simulink model "nonlinear_inverted_pendulum_simulation_direct"  (R2016b)
settings: Solver=ode15s  StartTime=0.0  StopTime=10.0  RelTol=1e-3
values from neighbouring files (symbols this model uses):
  A = sys.A    [LoopGain.m]    (also in dcontrold_dir.m = sys_d.A; main.m = [                   0,                                      ; simulation.m)
  B = sys.B    [LoopGain.m]    (also in dcontrold_dir.m = sys_d.B; main.m = [                   0; ( 3*Km*Vs)/(LinkMass*(LinkLength^2)*R; simulation.m)
  b_motor = 0    [main.m]
  C = sys.C    [LoopGain.m]    (also in dcontrold_dir.m = sys_d.C; main.m = [                   1,                                      ; simulation.m)
  g = 9.81    [main.m]
  J_total = 3.97396e-05    [InvPendModel.mat]    (also in main.m = 0.080955181411)
  K = place(A,B,Kp)    [dcontrold_dir.m]    (also in dcontrold_ind.m = place(A, B, desFbPoles); sysStateEstimatorFeedbackWithModel.m = Kaug(1:nStates))
  Kb = Km    (= 0.0265805280355)    [main.m]
  Km = Vs/kappa_id    (= 0.0265805280355)    [main.m]    (also in sysStateEstimatorFeedbackWithModel.m = Kaug(nStates + 1:end))
  L = place(A',C',Lp)'    [dcontrold_dir.m]    (also in dcontrold_ind.m = place(A', C', desObsPoles).')
  L_motor = 0.24E-3    (= 0.00024)    [main.m]
  LinkLength = 0.0508    [InvPendModel.mat]    (also in main.m = 0.07539)
  LinkMass = 0.045    [InvPendModel.mat]    (also in main.m = 42.73)
  N = 1 / (Cc * inv(eye(nStates)-sysCL.A) * Bc)    [analysis.m]
  R_motor = tau_id*Km^2 / J_total    (= 0.00175332528047)    [main.m]
  Ts = sys.Ts    [LoopGain.m]    (also in analysis.m = 1/Hz; main.m = T(tdx); simulation.m = 0.001; system_id_batch.m = 0.001)
  Vs = 12    [main.m]
libraries: cstblocks x1
settings Model: PauseTimes=1  Creator=pong0923  LastModifiedBy=pong0923
settings DataIOCC: ExternalInput=[m]

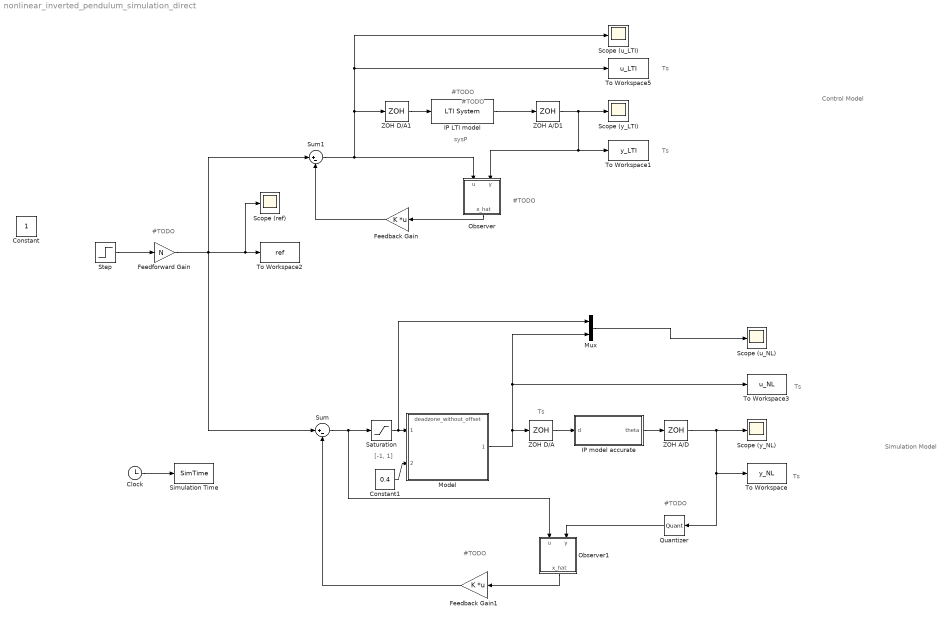
== system nonlinear_inverted_pendulum_simulation_direct ==
  note: Simulation Model
  note: Control Model
  note: #TODO
  note: #TODO
  note: sysP
  note: Ts
  note: Ts
  note: #TODO
  note: #TODO
  note: [-1, 1]
  note: Ts
  note: #TODO
  note: #TODO
  note: Ts
  note: Ts
  Clock : Clock
  Constant1 : Constant  Value=0.4
  Feedback Gain : Gain  Gain=K  Multiplication=Matrix(K*u)
  Feedback Gain1 : Gain  Gain=K  Multiplication=Matrix(K*u)
  Feedforward Gain : Gain  Gain=N
  IP LTI model : cstblocks/LTI System  sys=sysP  IC=[]
  IP model accurate : Subsystem
  Model : ModelReference  ModelNameDialog=deadzone_without_offset.slx  SimulationMode=Normal  ModelReferenceVersion=1.2
  Mux : Mux  Inputs=2
  Observer : Subsystem
  Observer1 : Subsystem
  Quantizer : Quantizer  QuantizationInterval=QzrLvl
  Saturation : Saturate  UpperLimit=1  LowerLimit=-1
  Scope (ref) : Scope
  Scope (u_LTI) : Scope
  Scope (u_NL) : Scope
  Scope (y_LTI) : Scope
  Scope (y_NL) : Scope
  Simulation Time : ToWorkspace  VariableName=SimTime  SampleTime=Ts
  Step : Step  After=0.2  SampleTime=Ts
  Sum : Sum  Inputs=|+-
  Sum1 : Sum  Inputs=|+-
  To Workspace : ToWorkspace  VariableName=y_NL  SaveFormat=Timeseries  SampleTime=Ts
  To Workspace1 : ToWorkspace  VariableName=y_LTI  SaveFormat=Timeseries  SampleTime=Ts
  To Workspace2 : ToWorkspace  VariableName=ref  SaveFormat=Timeseries  SampleTime=Ts
  To Workspace3 : ToWorkspace  VariableName=u_NL  SaveFormat=Timeseries  SampleTime=Ts
  To Workspace5 : ToWorkspace  VariableName=u_LTI  SaveFormat=Timeseries  SampleTime=Ts
  ZOH A/D : ZeroOrderHold  SampleTime=Ts
  ZOH A/D1 : ZeroOrderHold  SampleTime=Ts
  ZOH D/A : ZeroOrderHold  SampleTime=Ts
  ZOH D/A1 : ZeroOrderHold  SampleTime=Ts
  Constant : Constant  IOType=siggen
  wires:
  ZOH D/A/1 -> IP model accurate/1(d)
  IP model accurate/1(theta) -> ZOH A/D/1
  Clock/1 -> Simulation Time/1
  Sum/1 -> Observer1/1(u), Saturation/1
  Step/1 -> Feedforward Gain/1
  Feedforward Gain/1 -> Sum/1, Sum1/1, Scope (ref)/1, To Workspace2/1
  ZOH A/D/1 -> Quantizer/1, To Workspace/1, Scope (y_NL)/1
  Feedback Gain/1 -> Sum1/2
  Sum1/1 -> Observer/1(u), ZOH D/A1/1, To Workspace5/1, Scope (u_LTI)/1
  Feedback Gain1/1 -> Sum/2
  ZOH D/A1/1 -> IP LTI model/1
  ZOH A/D1/1 -> Observer/2(y), To Workspace1/1, Scope (y_LTI)/1
  IP LTI model/1 -> ZOH A/D1/1
  Observer/1(x_hat) -> Feedback Gain/1
  Quantizer/1 -> Observer1/2(y)
  Observer1/1(x_hat) -> Feedback Gain1/1
  Saturation/1 -> Mux/1, Model/1
  Model/1 -> Mux/2, To Workspace3/1, ZOH D/A/1
  Constant1/1 -> Model/2
  Mux/1 -> Scope (u_NL)/1

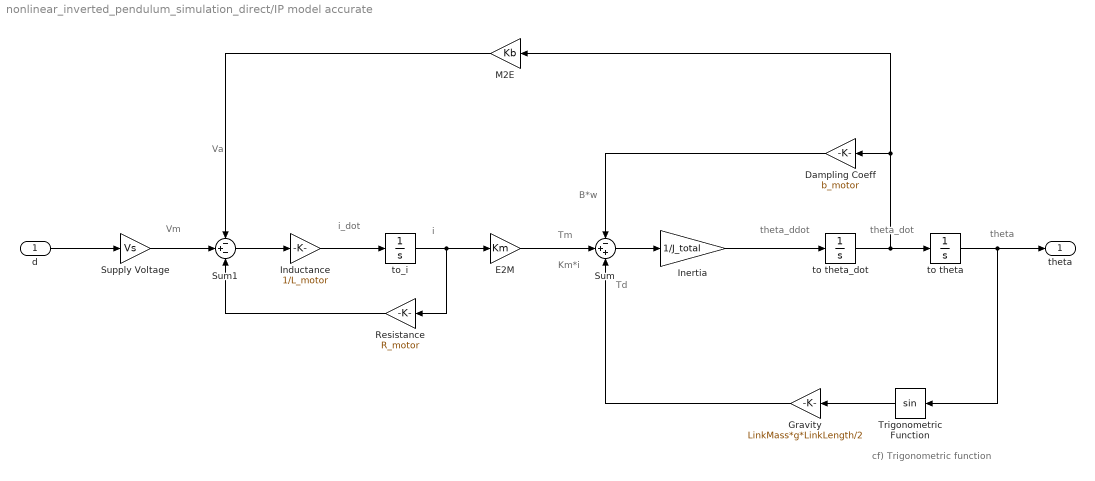
== system nonlinear_inverted_pendulum_simulation_direct/IP model accurate ==
  note: Va
  note: Vm
  note: i_dot
  note: B*w
  note: Td
  note: Km*i
  note: Tm
  note: i
  note: cf) Trigonometric
      | function
  note: theta_ddot
  note: theta
  note: theta_dot
  d : Inport
  Dampling Coeff : Gain  Gain=b_motor
  E2M : Gain  Gain=Km
  Gravity : Gain  Gain=LinkMass*g*LinkLength/2
  Inductance : Gain  Gain=1/L_motor
  Inertia : Gain  Gain=1/J_total
  M2E : Gain  Gain=Kb
  Resistance : Gain  Gain=R_motor
  Sum : Sum  Inputs=-++
  Sum1 : Sum  Inputs=-+-
  Supply Voltage : Gain  Gain=Vs
  Trigonometric Function : Trigonometry
  to theta : Integrator
  to theta_dot : Integrator
  to_i : Integrator
  theta : Outport
  wires:
  to theta_dot/1 -> to theta/1, M2E/1, Dampling Coeff/1
  to theta/1 -> Trigonometric Function/1, theta/1
  Trigonometric Function/1 -> Gravity/1
  E2M/1 -> Sum/2
  Dampling Coeff/1 -> Sum/1
  Gravity/1 -> Sum/3
  to_i/1 -> Resistance/1, E2M/1
  Resistance/1 -> Sum1/3
  d/1 -> Supply Voltage/1
  Supply Voltage/1 -> Sum1/2
  M2E/1 -> Sum1/1
  Sum1/1 -> Inductance/1
  Inductance/1 -> to_i/1
  Sum/1 -> Inertia/1
  Inertia/1 -> to theta_dot/1

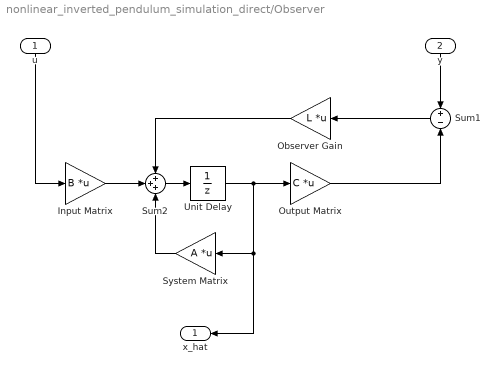
== system nonlinear_inverted_pendulum_simulation_direct/Observer ==
  u : Inport
  y : Inport  Port=2
  Input Matrix : Gain  Gain=B  Multiplication=Matrix(K*u)
  Observer Gain : Gain  Gain=L  Multiplication=Matrix(K*u)
  Output Matrix : Gain  Gain=C  Multiplication=Matrix(K*u)
  Sum1 : Sum  Inputs=+|-
  Sum2 : Sum  Inputs=+++
  System Matrix : Gain  Gain=A  Multiplication=Matrix(K*u)
  Unit Delay : UnitDelay  SampleTime=Ts
  x_hat : Outport
  wires:
  Sum1/1 -> Observer Gain/1
  System Matrix/1 -> Sum2/3
  Sum2/1 -> Unit Delay/1
  Output Matrix/1 -> Sum1/2
  Input Matrix/1 -> Sum2/2
  Observer Gain/1 -> Sum2/1
  u/1 -> Input Matrix/1
  Unit Delay/1 -> x_hat/1, System Matrix/1, Output Matrix/1
  y/1 -> Sum1/1

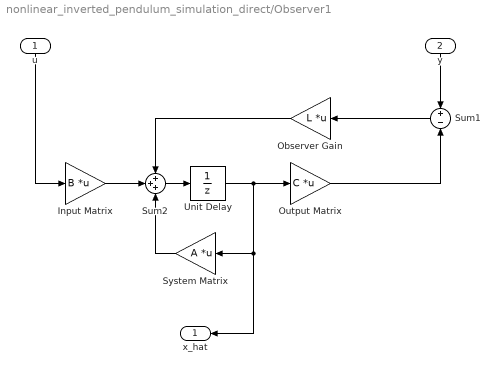
== system nonlinear_inverted_pendulum_simulation_direct/Observer1 ==
  u : Inport
  y : Inport  Port=2
  Input Matrix : Gain  Gain=B  Multiplication=Matrix(K*u)
  Observer Gain : Gain  Gain=L  Multiplication=Matrix(K*u)
  Output Matrix : Gain  Gain=C  Multiplication=Matrix(K*u)
  Sum1 : Sum  Inputs=+|-
  Sum2 : Sum  Inputs=+++
  System Matrix : Gain  Gain=A  Multiplication=Matrix(K*u)
  Unit Delay : UnitDelay  SampleTime=Ts
  x_hat : Outport
  wires:
  Sum1/1 -> Observer Gain/1
  System Matrix/1 -> Sum2/3
  Sum2/1 -> Unit Delay/1
  Output Matrix/1 -> Sum1/2
  Input Matrix/1 -> Sum2/2
  Observer Gain/1 -> Sum2/1
  u/1 -> Input Matrix/1
  Unit Delay/1 -> x_hat/1, System Matrix/1, Output Matrix/1
  y/1 -> Sum1/1
